simulink model "RL_pmsm"  (R2020b)
settings: Solver=ode45  StartTime=0.0  StopTime=200.0  RelTol=1e-3  EnableMultiTasking=on
undefined symbols (not defined in the file): Ts
libraries: powerlib x4, simulink x3, pid_lib x2, rllib x1
settings Model: Creator=The MathWorks, Inc.  LastModifiedBy=79006
settings DataIOCC: LimitDataPoints=on  SaveFormat=Array  ReturnWorkspaceOutputs=off  SignalLoggingName=logsOut
settings OptimizationCC: ExpressionDepthLimit=2147483647  InitFltsAndDblsToZero=on  LifeSpan=inf
settings DebuggingCC: SaveWithParameterizedLinksMsg=none  UnderspecifiedInitializationDetection=Classic  MergeDetectMultiDrivingBlocksExec=none  SignalResolutionControl=TryResolveAllWithWarning  MultiTaskDSMMsg=warning  FcnCallInpInsideContextMsg=warning  AllowSymbolicDim=off  StateNameClashWarn=warning  SFUnexpectedBacktrackingDiag=warning  SFNoUnconditionalDefaultTransitionDiag=warning  SFExecutionAtInitializationDiag=none  ArithmeticOperatorsInVariantConditions=warning
settings HardwareCC: ProdBitPerPointer=32  ProdBitPerSizeT=32  ProdBitPerPtrDiffT=32  ProdLargestAtomicFloat=None  ProdIntDivRoundTo=Undefined  ProdEndianess=Unspecified  ProdWordSize=32  ProdHWDeviceType=Specified
settings ModelReferenceCC: PropagateSignalLabelsOutOfModel=off
settings SFSimCC: SimUseLocalCustomCode=off
settings RTWCC: RTWUseLocalCustomCode=off
settings CodeAppCC: StateflowObjectComments=on
settings GRTTargetCC: TargetFcnLib=ansi_tfl_tmw.mat  TargetLangStandard=C89/C90 (ANSI)  CombineOutputUpdateFcns=off  GRTInterface=on
settings ConfigComp: CovMetricSettings=dw  CovSaveCumulativeToWorkspaceVar=on  CovSaveSingleToWorkspaceVar=on  CovExternalEMLEnable=off

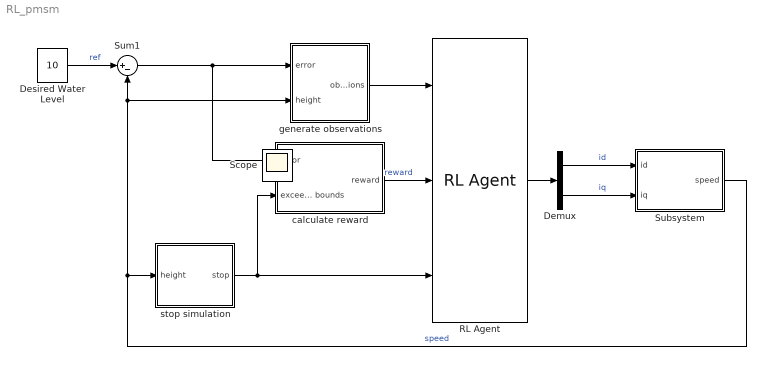
== system RL_pmsm ==
  Demux : Demux  Outputs=2
  Desired Water Level : Constant  Value=10
  RL Agent : rllib/RL Agent  Agent=agent  ProvideReward=on  ProvideIsDone=on  ProvideCumRwd=off  TreatAsDirectFeedthrough=on  CollectLoggedSignals=on  CollectModelStates=on
      settings: SourceProductName=Reinforcement Learning
  Subsystem : Subsystem
  Sum1 : Sum  Inputs=|+-  SaturateOnIntegerOverflow=on
  calculate reward : Subsystem
  generate observations : Subsystem
  stop simulation : Subsystem
  Scope : Scope
  wires:
  Desired Water Level/1 -> Sum1/1  "ref"
  Sum1/1 -> calculate reward/1(error), generate observations/1(error)
  Subsystem/1(speed) -> stop simulation/1(height), generate observations/2(height), Sum1/2  "speed"
  RL Agent/1 -> Demux/1
  stop simulation/1(stop) -> RL Agent/3, calculate reward/2(exceeds bounds)
  calculate reward/1(reward) -> RL Agent/2  "reward"
  generate observations/1(observations) -> RL Agent/1
  Demux/1 -> Subsystem/1(id)  "id"
  Demux/2 -> Subsystem/2(iq)  "iq"

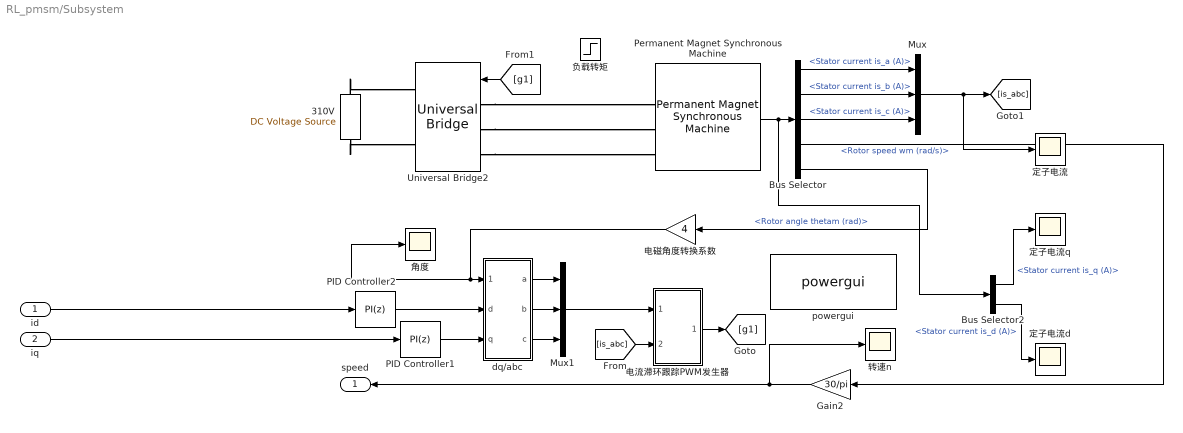
== system RL_pmsm/Subsystem ==
  id : Inport
  iq : Inport  Port=2
  310V : powerlib/Electrical Sources/DC Voltage Source  Amplitude=310  Measurements=None
  Bus Selector : BusSelector  OutputSignals=Stator current is_a (A),Stator current is_b (A),Stator current is_c (A),Rotor speed wm (rad/s),Rotor angle thetam (rad)
  Bus Selector2 : BusSelector  OutputSignals=Stator current is_q (A),Stator current is_d (A)
  Gain2 : Gain  Gain=30/pi
  Mux : Mux  Inputs=3
  Mux1 : Mux  Inputs=3
  PID Controller1 : pid_lib/PID Controller  Controller=PI  Form=Parallel  TimeDomain=Discrete-time  UseExternalTs=off  SampleTime=Ts  IntegratorMethod=Forward Euler  FilterMethod=Forward Euler  ControllerParametersSource=internal  P=1  I=0  D=0  UseFilter=on  N=100  TunerSelectOption=Transfer Function Based (PID Tuner App)  InitialConditionSource=internal  InitialConditionForIntegrator=0  InitialConditionForFilter=0  DifferentiatorICPrevScaledInput=0  ExternalReset=none  TrackingMode=off  Kt=1  LimitOutput=off  SatLimitsSource=internal  UpperSaturationLimit=200  LowerSaturationLimit=-inf  LinearizeAsGain=on  AntiWindupMode=none  Kb=1  POutMin=[]  POutMax=[]  IOutMin=[]  IOutMax=[]  DOutMin=[]  DOutMax=[]  NOutMin=[]  NOutMax=[]  SumOutMin=[]  SumOutMax=[]  SaturationOutMin=[]  SaturationOutMax=[]  PParamMin=[]  PParamMax=[]  IParamMin=[]  IParamMax=[]  DParamMin=[]  DParamMax=[]  NParamMin=[]  NParamMax=[]  KbParamMin=[]  KbParamMax=[]  KtParamMin=[]  KtParamMax=[]  KbOutMin=[]  KbOutMax=[]  KtOutMin=[]  KtOutMax=[]  IntegratorOutMin=[]  IntegratorOutMax=[]  FilterOutMin=[]  FilterOutMax=[]  SumI1OutMin=[]  SumI1OutMax=[]  SumI2OutMin=[]  SumI2OutMax=[]  SumI3OutMin=[]  SumI3OutMax=[]  SumI4OutMin=[]  SumI4OutMax=[]  SumDOutMin=[]  SumDOutMax=[]  DifferentiatorOutMin=[]  DifferentiatorOutMax=[]  FilterDiffOutCoefMin=[]  FilterDiffOutCoefMax=[]  ReciprocalOutMin=[]  ReciprocalOutMax=[]  SumDenOutMin=[]  SumDenOutMax=[]  SumNumOutMin=[]  SumNumOutMax=[]  DivideOutMin=[]  DivideOutMax=[]  UdiffTsProdOutMin=[]  UdiffTsProdOutMax=[]  NTsProdOutMin=[]  NTsProdOutMax=[]  UintegralTsProdOutMin=[]  UintegralTsProdOutMax=[]  UngainTsProdOutMin=[]  UngainTsProdOutMax=[]  IntegratorContinuousStateAttributes=''  IntegratorStateMustResolveToSignalObject=off  IntegratorRTWStateStorageClass=Auto  FilterContinuousStateAttributes=''  FilterStateMustResolveToSignalObject=off  FilterRTWStateStorageClass=Auto  ParallelPVariant=InternalParameters  IdealPVariant=Disabled  IVariant=InternalParameters  DVariant=Disabled  IntegratorVariant=Discrete  SatVariant=Disabled  AWVariant=Passthrough  PCopyVariant=Disabled  TRVariant=Disabled  FdbkBlocksVariant=Forward  IdealPFdbkVariant=Disabled  SatFdbkVariant=Disabled  DerivativeFilterVariant=Disabled  NVariant=Disabled  NCopyVariant=Disabled_SignalSpec  FilterICVariant=Disabled  IntegratorICVariant=InternalICs  ExternalResetVariant=Disabled  TRSumVariant=Passthrough  SumFdbkVariant=Disabled  SumVariant=Sum_PI  TsampFilterVariant=InternalTs  TsampNgainVariant=Passthrough  TsampIntegralVariant=Passthrough  ExternalSaturationOutDataTypeStr=Inherit: Same as second input
  PID Controller2 : pid_lib/PID Controller  Controller=PI  Form=Parallel  TimeDomain=Discrete-time  UseExternalTs=off  SampleTime=Ts  IntegratorMethod=Forward Euler  FilterMethod=Forward Euler  ControllerParametersSource=internal  P=1  I=0  D=0  UseFilter=on  N=100  TunerSelectOption=Transfer Function Based (PID Tuner App)  InitialConditionSource=internal  InitialConditionForIntegrator=0  InitialConditionForFilter=0  DifferentiatorICPrevScaledInput=0  ExternalReset=none  TrackingMode=off  Kt=1  LimitOutput=off  SatLimitsSource=internal  UpperSaturationLimit=200  LowerSaturationLimit=-inf  LinearizeAsGain=on  AntiWindupMode=none  Kb=1  POutMin=[]  POutMax=[]  IOutMin=[]  IOutMax=[]  DOutMin=[]  DOutMax=[]  NOutMin=[]  NOutMax=[]  SumOutMin=[]  SumOutMax=[]  SaturationOutMin=[]  SaturationOutMax=[]  PParamMin=[]  PParamMax=[]  IParamMin=[]  IParamMax=[]  DParamMin=[]  DParamMax=[]  NParamMin=[]  NParamMax=[]  KbParamMin=[]  KbParamMax=[]  KtParamMin=[]  KtParamMax=[]  KbOutMin=[]  KbOutMax=[]  KtOutMin=[]  KtOutMax=[]  IntegratorOutMin=[]  IntegratorOutMax=[]  FilterOutMin=[]  FilterOutMax=[]  SumI1OutMin=[]  SumI1OutMax=[]  SumI2OutMin=[]  SumI2OutMax=[]  SumI3OutMin=[]  SumI3OutMax=[]  SumI4OutMin=[]  SumI4OutMax=[]  SumDOutMin=[]  SumDOutMax=[]  DifferentiatorOutMin=[]  DifferentiatorOutMax=[]  FilterDiffOutCoefMin=[]  FilterDiffOutCoefMax=[]  ReciprocalOutMin=[]  ReciprocalOutMax=[]  SumDenOutMin=[]  SumDenOutMax=[]  SumNumOutMin=[]  SumNumOutMax=[]  DivideOutMin=[]  DivideOutMax=[]  UdiffTsProdOutMin=[]  UdiffTsProdOutMax=[]  NTsProdOutMin=[]  NTsProdOutMax=[]  UintegralTsProdOutMin=[]  UintegralTsProdOutMax=[]  UngainTsProdOutMin=[]  UngainTsProdOutMax=[]  IntegratorContinuousStateAttributes=''  IntegratorStateMustResolveToSignalObject=off  IntegratorRTWStateStorageClass=Auto  FilterContinuousStateAttributes=''  FilterStateMustResolveToSignalObject=off  FilterRTWStateStorageClass=Auto  ParallelPVariant=InternalParameters  IdealPVariant=Disabled  IVariant=InternalParameters  DVariant=Disabled  IntegratorVariant=Discrete  SatVariant=Disabled  AWVariant=Passthrough  PCopyVariant=Disabled  TRVariant=Disabled  FdbkBlocksVariant=Forward  IdealPFdbkVariant=Disabled  SatFdbkVariant=Disabled  DerivativeFilterVariant=Disabled  NVariant=Disabled  NCopyVariant=Disabled_SignalSpec  FilterICVariant=Disabled  IntegratorICVariant=InternalICs  ExternalResetVariant=Disabled  TRSumVariant=Passthrough  SumFdbkVariant=Disabled  SumVariant=Sum_PI  TsampFilterVariant=InternalTs  TsampNgainVariant=Passthrough  TsampIntegralVariant=Passthrough  ExternalSaturationOutDataTypeStr=Inherit: Same as second input
  Permanent Magnet Synchronous Machine : powerlib/Machines/Permanent Magnet Synchronous Machine  NbPhases=3  FluxDistribution=Sinusoidal  RotorType=Salient-pole  MechanicalLoad=Torque Tm  PresetModel=No  ShowDetailedParameters=on  MeasurementBus=off  Resistance=2.785  Inductance=8.5e-3  dqInductances=[0.0085 0.0085]  La=0.02682  MachineConstant=Flux linkage established by magnets (V.s)  Flux=0.175  VoltageCst=126.966  TorqueCst=1.05  Flat=120  Mechanical=[0.001 0.008 4 0]  PolePairs=2  InitialConditions=[0,0, 0,0]  InitialConditions5ph=[0 0 0 0 0 0]  RefAngle=Aligned with phase A axis (original Park)  IterativeDiscreteModel=Trapezoidal non iterative  TsBlock=-1  TsPowergui=0
  Universal Bridge2 : powerlib/Power Electronics/Universal Bridge  Arms=3  SnubberResistance=1e5  SnubberCapacitance=inf  Device=IGBT / Diodes  Ron=1e-3  Lon=0  ForwardVoltages="[  0  0  ]"  ForwardVoltage=0  GTOparameters=[ 10e-6 , 20e-6 ]  IGBTparameters=[ 1e-6 , 2e-6 ]  Measurements=None  Measurements_2=None  converterType=Rectifier
  dq/abc : Subsystem
  powergui : powerlib/powergui  SimulationMode=Discrete  SampleTime=Ts  frequency=50  Iterations=50  frequencyindice=0  Pbase=100e6  ErrMax=1e-4  UnitsV=kV  UnitsW=MW  buscounter=0  FunctionMessages=off  echomessages=off  EnableUseOfTLC=off  CurrentSourceSwitches=off  DisableSnubberDevices=off  DisableRonSwitches=off  DisableVfSwitches=off  DisplayEquations=off  AutomaticDiscreteSolvers=off  SolverType=Tustin/Backward Euler (TBE)  Interpol=off  ExternalGateDelay=off  methode=off  Ts=100  x0status=zero  SPID=on  SwTol=0  HookPort=off  NonlinearTolerance=1e-4  nMaxIteration=100  ContinueOnMaxIteration=off  RestoreLinks=warning  ResistiveCurrentMeasurement=off  Frange=[0:2:500]  Ylog=off  Xlog=on  ShowGrid=off  save=off  variable=ZData  structure=0  ZoomFFT=on  StartTime=0.0  cycles=1  DisplayStyle=1  fundamental=60  FreqAxis=off  MaxFrequency=1000  frequencyindicesteady=1  RmsSteady=1  display=off
  定子电流 : Scope
  定子电流d : Scope
  定子电流q : Scope
  电流滞环跟踪PWM发生器 : Subsystem
  电磁角度转换系数 : Gain  Gain=4
  角度 : Scope
  负载转矩 : Step  Time=0.02  Before=4  After=10  SampleTime=0
  转速n : Scope
  speed : Outport
  wires:
  电流滞环跟踪PWM发生器/1(pulse) -> [g1]
  Permanent Magnet Synchronous Machine/1 -> Bus Selector2/1, Bus Selector/1
  dq/abc/3(c) -> Mux1/3
  dq/abc/1(a) -> Mux1/1
  PID Controller2/1 -> dq/abc/2(d)
  Bus Selector/1 -> Mux/1  "<Stator current is_a (A)>"
  [is_abc] -> 电流滞环跟踪PWM发生器/2(Iabc)
  Bus Selector/3 -> Mux/3  "<Stator current is_c (A)>"
  Bus Selector/4 -> Gain2/1  "<Rotor speed wm (rad/s)>"
  Bus Selector2/2 -> 定子电流d/1  "<Stator current is_d (A)>"
  Mux1/1 -> 电流滞环跟踪PWM发生器/1(Iabc*)
  Gain2/1 -> speed/1, 转速n/1
  dq/abc/2(b) -> Mux1/2
  Bus Selector/5 -> 电磁角度转换系数/1  "<Rotor angle thetam (rad)>"
  电磁角度转换系数/1 -> 角度/1, dq/abc/1(theta)
  id/1 -> PID Controller2/1
  Mux/1 -> 定子电流/1, [is_abc]
  Bus Selector/2 -> Mux/2  "<Stator current is_b (A)>"
  [g1] -> Universal Bridge2/1
  Bus Selector2/1 -> 定子电流q/1  "<Stator current is_q (A)>"
  iq/1 -> PID Controller1/1
  PID Controller1/1 -> dq/abc/3(q)
  connections:
  310V/RConn1 -- Universal Bridge2/RConn1
  Universal Bridge2/LConn3 -- Permanent Magnet Synchronous Machine/LConn3
  Universal Bridge2/LConn1 -- Permanent Magnet Synchronous Machine/LConn1
  310V/LConn1 -- Universal Bridge2/RConn2
  Universal Bridge2/LConn2 -- Permanent Magnet Synchronous Machine/LConn2

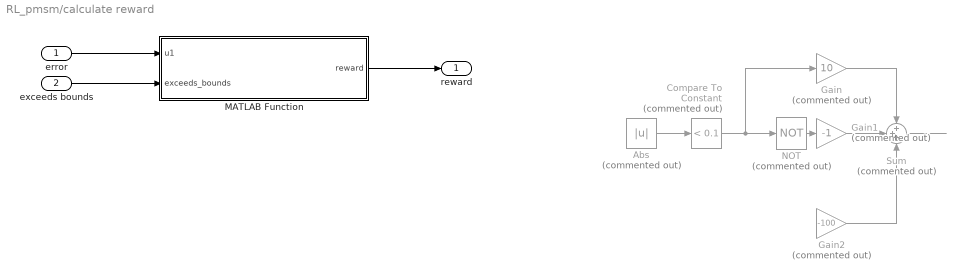
== system RL_pmsm/calculate reward ==
  error : Inport
  exceeds bounds : Inport  Port=2
  Abs : Abs  Commented=on
  Compare To Constant : simulink/Logic and Bit Operations/Compare To Constant  Commented=on  relop=<  const=0.1  OutDataTypeStr=boolean
  Gain : Gain  Commented=on  Gain=10
  Gain1 : Gain  Commented=on  Gain=-1
  Gain2 : Gain  Commented=on  Gain=-100
  MATLAB Function : MATLAB Function  TreatAsAtomicUnit=on
  NOT : Logic  Commented=on  Operator=NOT  IconShape=distinctive  AllPortsSameDT=off  OutDataTypeStr=boolean
  Sum : Sum  Commented=on  Inputs=+++  OutDataTypeStr=double
  reward : Outport  VectorParamsAs1DForOutWhenUnconnected=off
  wires:
  NOT/1 -> Gain1/1
  ? -> Abs/1
  ? -> Gain2/1
  Gain2/1 -> Sum/3
  Gain1/1 -> Sum/2
  Compare To Constant/1 -> NOT/1, Gain/1
  Gain/1 -> Sum/1
  Sum/1 -> ?
  Abs/1 -> Compare To Constant/1
  exceeds bounds/1 -> MATLAB Function/2(exceeds_bounds)
  error/1 -> MATLAB Function/1(u1)
  MATLAB Function/1(reward) -> reward/1

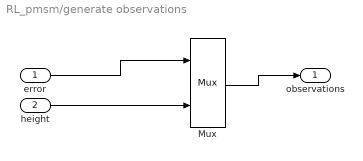
== system RL_pmsm/generate observations ==
  error : Inport
  height : Inport  Port=2
  Mux : Mux  Inputs=2
  observations : Outport  VectorParamsAs1DForOutWhenUnconnected=off
  wires:
  error/1 -> Mux/1
  Mux/1 -> observations/1
  height/1 -> Mux/2

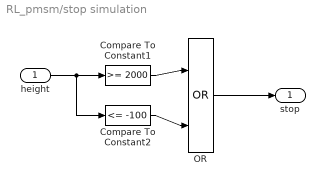
== system RL_pmsm/stop simulation ==
  height : Inport
  Compare To Constant1 : simulink/Logic and Bit Operations/Compare To Constant  relop=>=  const=2000  OutDataTypeStr=boolean
  Compare To Constant2 : simulink/Logic and Bit Operations/Compare To Constant  relop=<=  const=-100  OutDataTypeStr=boolean
  OR : Logic  Operator=OR  IconShape=distinctive  AllPortsSameDT=off  OutDataTypeStr=boolean
  stop : Outport  VectorParamsAs1DForOutWhenUnconnected=off
  wires:
  height/1 -> Compare To Constant2/1, Compare To Constant1/1
  Compare To Constant1/1 -> OR/1
  OR/1 -> stop/1
  Compare To Constant2/1 -> OR/2

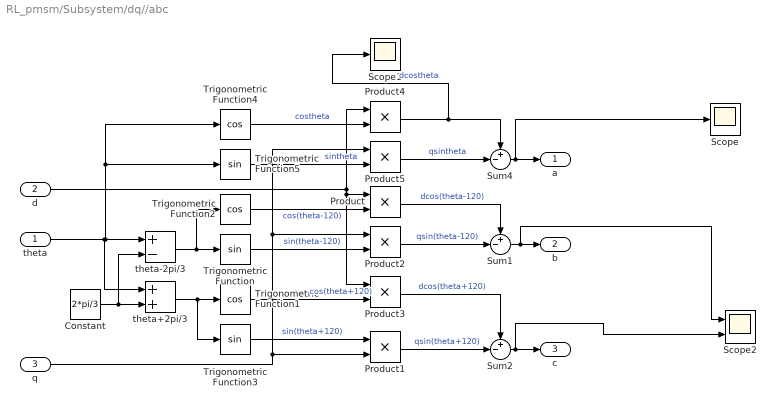
== system RL_pmsm/Subsystem/dq//abc ==
  theta : Inport
  d : Inport  Port=2
  q : Inport  Port=3
  Constant : Constant  Value=2*pi/3
  Product{,1..5} (6 alike) : Product
  Scope : Scope
  Scope1 : Scope
  Scope2 : Scope  NumInputPorts=2
  Sum1 : Sum  Inputs=+-|
  Sum2 : Sum  Inputs=+-|
  Sum4 : Sum  Inputs=+-|
  Trigonometric Function : Trigonometry
  Trigonometric Function1 : Trigonometry  Operator=cos
  Trigonometric Function2 : Trigonometry  Operator=cos
  Trigonometric Function3 : Trigonometry
  Trigonometric Function4 : Trigonometry  Operator=cos
  Trigonometric Function5 : Trigonometry
  theta+2pi/3 : Sum
  theta-2pi/3 : Sum  Inputs=+-
  a : Outport  VectorParamsAs1DForOutWhenUnconnected=off
  b : Outport  Port=2  VectorParamsAs1DForOutWhenUnconnected=off
  c : Outport  Port=3  VectorParamsAs1DForOutWhenUnconnected=off
  wires:
  Trigonometric Function5/1 -> Product5/2  "sintheta"
  Product/1 -> Sum1/1  "dcos(theta-120)"
  Trigonometric Function1/1 -> Product3/2  "cos(theta+120)"
  Product3/1 -> Sum2/1  "dcos(theta+120)"
  d/1 -> Product/1, Product3/1, Product4/1
  Constant/1 -> theta+2pi/3/2, theta-2pi/3/2
  theta/1 -> Trigonometric Function4/1, Trigonometric Function5/1, theta-2pi/3/1, theta+2pi/3/1
  theta+2pi/3/1 -> Trigonometric Function3/1, Trigonometric Function1/1
  q/1 -> Product5/1, Product2/1, Product1/2
  Trigonometric Function/1 -> Product2/2  "sin(theta-120)"
  Product4/1 -> Scope1/1, Sum4/1  "dcostheta"
  Product5/1 -> Sum4/2  "qsintheta"
  theta-2pi/3/1 -> Trigonometric Function2/1, Trigonometric Function/1
  Product1/1 -> Sum2/2  "qsin(theta+120)"
  Trigonometric Function2/1 -> Product/2  "cos(theta-120)"
  Sum4/1 -> Scope/1, a/1
  Sum1/1 -> Scope2/1, b/1
  Trigonometric Function4/1 -> Product4/2  "costheta"
  Trigonometric Function3/1 -> Product1/1  "sin(theta+120)"
  Product2/1 -> Sum1/2  "qsin(theta-120)"
  Sum2/1 -> Scope2/2, c/1

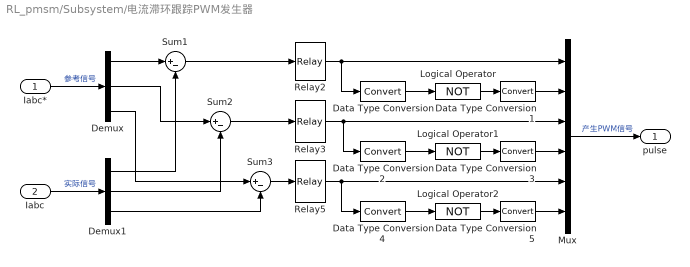
== system RL_pmsm/Subsystem/电流滞环跟踪PWM发生器 ==
  Iabc* : Inport
  Iabc : Inport  Port=2
  Data Type Conversion{,1..5} (6 alike) : DataTypeConversion
  Demux : Demux  Outputs=3
  Demux1 : Demux  Outputs=3
  Logical Operator : Logic  Operator=NOT  Inputs=1  AllPortsSameDT=off
  Logical Operator1 : Logic  Operator=NOT  Inputs=1  AllPortsSameDT=off
  Logical Operator2 : Logic  Operator=NOT  Inputs=1  AllPortsSameDT=off
  Mux : Mux  Inputs=6
  Relay2 : Relay  OnSwitchValue=0.1  OffSwitchValue=-0.1  ZeroCross=off
  Relay3 : Relay  OnSwitchValue=0.1  OffSwitchValue=-0.1  ZeroCross=off
  Relay5 : Relay  OnSwitchValue=0.1  OffSwitchValue=-0.1  ZeroCross=off
  Sum1 : Sum  Inputs=|+-
  Sum2 : Sum  Inputs=|+-
  Sum3 : Sum  Inputs=|+-
  pulse : Outport  VectorParamsAs1DForOutWhenUnconnected=off
  wires:
  Relay2/1 -> Data Type Conversion/1, Mux/1
  Data Type Conversion/1 -> Logical Operator/1
  Logical Operator/1 -> Data Type Conversion1/1
  Data Type Conversion1/1 -> Mux/2
  Mux/1 -> pulse/1  "产生PWM信号"
  Sum1/1 -> Relay2/1
  Demux/1 -> Sum1/1
  Demux1/3 -> Sum3/2
  Iabc/1 -> Demux1/1  "实际信号"
  Iabc*/1 -> Demux/1  "参考信号"
  Sum2/1 -> Relay3/1
  Logical Operator1/1 -> Data Type Conversion3/1
  Data Type Conversion3/1 -> Mux/4
  Data Type Conversion2/1 -> Logical Operator1/1
  Relay3/1 -> Data Type Conversion2/1, Mux/3
  Logical Operator2/1 -> Data Type Conversion5/1
  Data Type Conversion5/1 -> Mux/6
  Data Type Conversion4/1 -> Logical Operator2/1
  Relay5/1 -> Data Type Conversion4/1, Mux/5
  Sum3/1 -> Relay5/1
  Demux/2 -> Sum2/1
  Demux1/1 -> Sum1/2
  Demux1/2 -> Sum2/2
  Demux/3 -> Sum3/1

== matlab function RL_pmsm/calculate reward/MATLAB Function ==
  data: u1 input; reward output; exceeds_bounds input
function reward = fcn(u1,exceeds_bounds)
reward = 0;
u1 = abs(u1);
if(u1 < 10)
    reward = u1;
else
    reward = -1 * u1;
end
reward = reward +  exceeds_bounds*1000;
